simulink model "diag_bloqu"  (R2024a)
settings: Solver=VariableStepAuto  StartTime=0.0  StopTime=30  RelTol=1e-3
settings Model: Creator=Adriana  LastModifiedBy=Juan
settings ModelReferenceCC: EnableRefExpFcnMdlSchedulingChecks=on
settings RTWCC: GPUComputeCapability=3.5

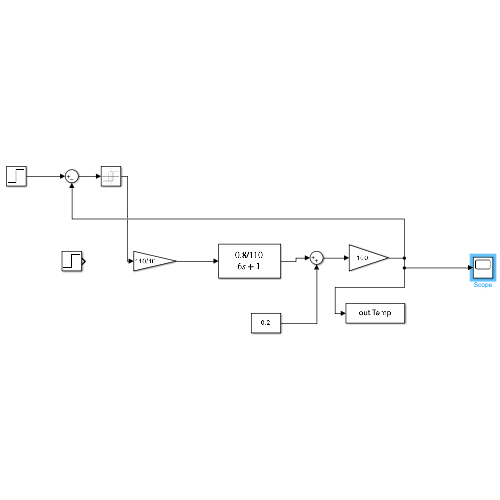
[thumbnail: Simulink's stored preview of the top-level diagram]
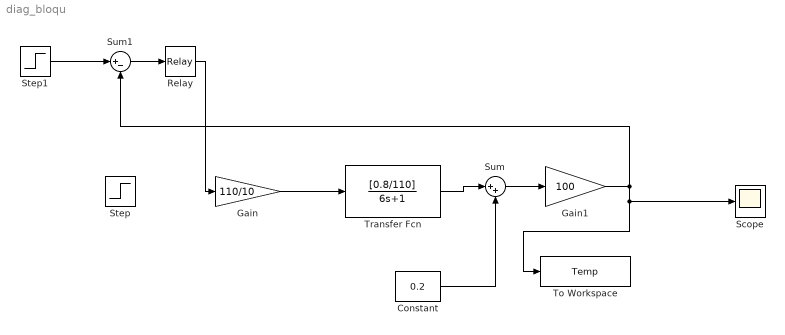
== system diag_bloqu ==
  Constant : Constant  Value=0.2
  Gain : Gain  Gain=110/10
  Gain1 : Gain  Gain=100
  Relay : Relay  OnSwitchValue=1  OffSwitchValue=-1  OnOutputValue=10
  Scope : Scope
  Step : Step  Time=0  After=10  SampleTime=0
  Step1 : Step  Time=0  After=60  SampleTime=0
  Sum : Sum  Inputs=|++
  Sum1 : Sum  Inputs=|+-
  To Workspace : ToWorkspace  VariableName=Temp  SaveFormat=Timeseries  SampleTime=-1
  Transfer Fcn : TransferFcn  Numerator=[0.8/110]  Denominator=[6 1]
  wires:
  Gain/1 -> Transfer Fcn/1
  Transfer Fcn/1 -> Sum/1
  Constant/1 -> Sum/2
  Sum/1 -> Gain1/1
  Step1/1 -> Sum1/1
  Sum1/1 -> Relay/1
  Gain1/1 -> Sum1/2, Scope/1, To Workspace/1
  Relay/1 -> Gain/1
